simulink model "asgm2_exc2"  (R2024a)
settings: Solver=VariableStepAuto  StartTime=0.0  StopTime=20  RelTol=1e-3
undefined symbols (not defined in the file): A, B, C, E, F, Fy, H, K, T
settings Model: Creator=HIEDA  LastModifiedBy=HIEDA

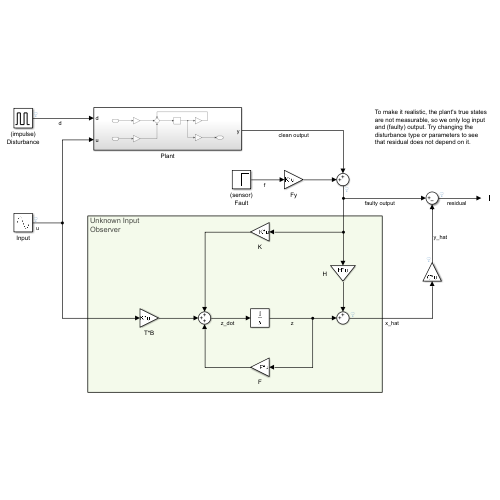
[thumbnail: Simulink's stored preview of the top-level diagram]
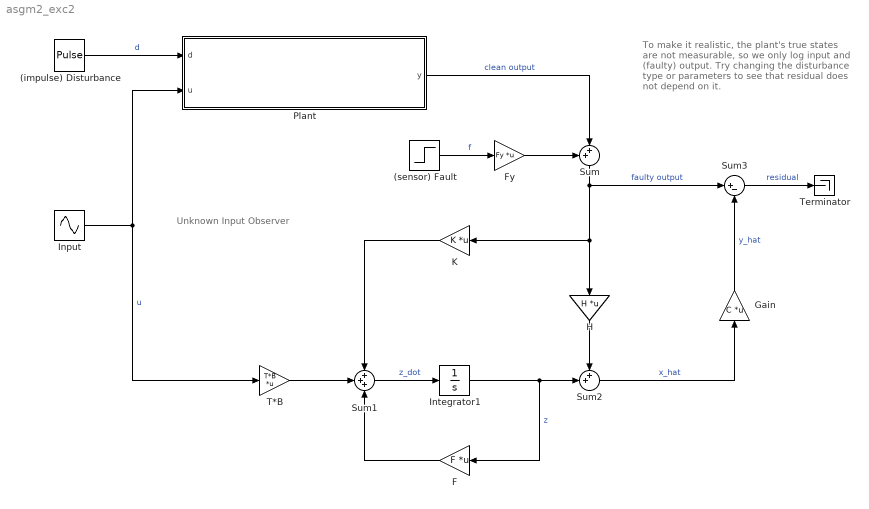
== system asgm2_exc2 ==
  note: To make it realistic, the plant's true states are not measurable, so we only log input and (faulty) output. Try changing the disturbance type or parameters to see that residual does not depend on it.
  note: Unknown Input
      | Observer
  (impulse) Disturbance : DiscretePulseGenerator  PulseType=Time based  Amplitude=0.2  Period=10  PulseWidth=25  PhaseDelay=pi/4
  (sensor) Fault : Step  Time=10  After=1.17  SampleTime=0
  F : Gain  Gain=F  Multiplication=Matrix(K*u)
  Fy : Gain  Gain=Fy  Multiplication=Matrix(K*u)
  Gain : Gain  Gain=C  Multiplication=Matrix(K*u)
  H : Gain  Gain=H  Multiplication=Matrix(K*u)
  Input : Sin  SampleTime=0
  Integrator1 : Integrator  InitialCondition=zeros(4,1)
  K : Gain  Gain=K  Multiplication=Matrix(K*u)
  Plant : Subsystem
  Sum : Sum  Inputs=++|
  Sum1 : Sum  Inputs=+++
  Sum2 : Sum  Inputs=++|
  Sum3 : Sum  Inputs=|+-
  T*B : Gain  Gain=T*B  Multiplication=Matrix(K*u)
  Terminator : Terminator
  wires:
  K/1 -> Sum1/1
  T*B/1 -> Sum1/2
  Sum1/1 -> Integrator1/1  "z_dot"
  Integrator1/1 -> F/1, Sum2/2  "z"
  H/1 -> Sum2/1
  F/1 -> Sum1/3
  Sum2/1 -> Gain/1  "x_hat"
  Sum/1 -> Sum3/1, K/1, H/1  "faulty output"
  Input/1 -> Plant/2(u), T*B/1  "u"
  (sensor) Fault/1 -> Fy/1  "f"
  Fy/1 -> Sum/1
  Plant/1(y) -> Sum/2  "clean output"
  Gain/1 -> Sum3/2  "y_hat"
  Sum3/1 -> Terminator/1  "residual"
  (impulse) Disturbance/1 -> Plant/1(d)  "d"

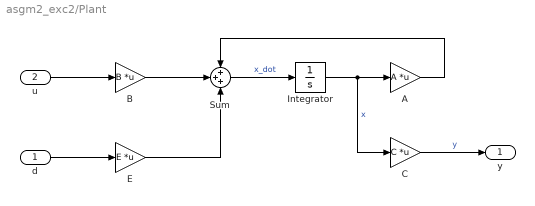
== system asgm2_exc2/Plant ==
  d : Inport
  u : Inport  Port=2
  A : Gain  Gain=A  Multiplication=Matrix(K*u)
  B : Gain  Gain=B  Multiplication=Matrix(K*u)
  C : Gain  Gain=C  Multiplication=Matrix(K*u)
  E : Gain  Gain=E  Multiplication=Matrix(K*u)
  Integrator : Integrator  InitialCondition=zeros(4,1)
  Sum : Sum  Inputs=+++
  y : Outport
  wires:
  Integrator/1 -> C/1, A/1  "x"
  u/1 -> B/1
  B/1 -> Sum/2
  Sum/1 -> Integrator/1  "x_dot"
  A/1 -> Sum/1
  C/1 -> y/1  "y"
  d/1 -> E/1
  E/1 -> Sum/3
